simulink model "rull_stamp_hiv_modell"  (R2022a)
settings: Solver=VariableStepAuto  StartTime=0.0  StopTime=30  RelTol=1e-3
values from neighbouring files (symbols this model uses):
  A_topp = 0.286615    [Modell_verdier.m]
  B_r_t = 0.000799434    [Modell_verdier.m]
  B_s_f = 0.002833197    [Modell_verdier.m]
  B_s_t = 0.000183411    [Modell_verdier.m]
  C_D = 1.28    [Modell_verdier.m]
  Fb = 226    [Modell_verdier.m]
  g = 9.81    [Modell_verdier.m]
  I_rull = 1.28294    [Modell_verdier.m]
  I_stamp = 1.29837    [Modell_verdier.m]
  masse = 22.49    [Modell_verdier.m]
  phi_motor_rull = deg2rad(90-61.7)    [Modell_verdier.m]
  r_Fb = 0.036    [Modell_verdier.m]
  r_motor_rull = 0.277    [Modell_verdier.m]
  r_motor_stamp = 0.269    [Modell_verdier.m]
  tetthet_vann = 1000    [Modell_verdier.m]
  theta_motor_stamp = deg2rad(90-60.8)    [Modell_verdier.m]
libraries: simulink_extras x6
settings Model: Creator=andre  LastModifiedBy=andre

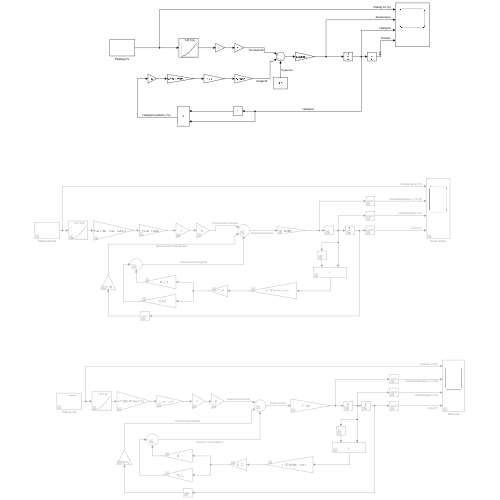
[thumbnail: Simulink's stored preview of the top-level diagram]
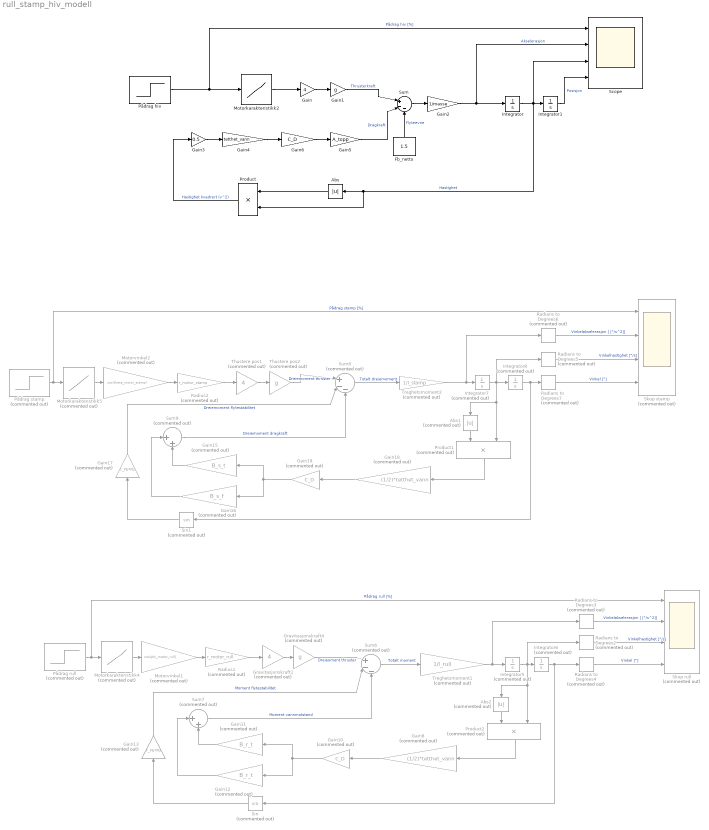
== system rull_stamp_hiv_modell ==
  Abs : Abs  SaturateOnIntegerOverflow=off
  Abs1 : Abs  Commented=on  SaturateOnIntegerOverflow=off
  Abs2 : Abs  Commented=on  SaturateOnIntegerOverflow=off
  Fb_netto : Constant  Value=1.5
  Gain : Gain  Gain=4
  Gain1 : Gain  Gain=g
  Gain10 : Gain  Commented=on  Gain=C_D
  Gain11 : Gain  Commented=on  Gain=B_r_t
  Gain12 : Gain  Commented=on  Gain=B_r_t
  Gain13 : Gain  Commented=on  Gain=r_Fb*Fb
  Gain15 : Gain  Commented=on  Gain=B_s_t
  Gain16 : Gain  Commented=on  Gain=B_s_f
  Gain17 : Gain  Commented=on  Gain=r_Fb*Fb
  Gain18 : Gain  Commented=on  Gain=(1/2)*tetthet_vann
  Gain19 : Gain  Commented=on  Gain=C_D
  Gain2 : Gain  Gain=1/masse
  Gain3 : Gain  Gain=0.5
  Gain4 : Gain  Gain=tetthet_vann
  Gain5 : Gain  Gain=A_topp
  Gain6 : Gain  Gain=C_D
  Gain8 : Gain  Commented=on  Gain=(1/2)*tetthet_vann
  Gravitasjonskraft1 : Gain  Commented=on  Gain=4
  Gravitasjonskraft4 : Gain  Commented=on  Gain=g
  Integrator : Integrator
  Integrator1 : Integrator  InitialCondition=0.5
  Integrator5 : Integrator  Commented=on
  Integrator6 : Integrator  Commented=on  InitialCondition=pi/4
  Integrator7 : Integrator  Commented=on
  Integrator8 : Integrator  Commented=on  InitialCondition=pi/4
  Motorkarakteristikk2 : Lookup_n-D  NumberOfTableDimensions=1  BreakpointsForDimension1="[0   12.5000   25.0000   37.5000   50.0000   62.5000   75.0000   87.5000  100.0000]"  Table=[0 0.1403 0.2807 0.5874 0.8942 1.3908 1.8874 2.3507 2.8140]  InternalRulePriority=Speed  RndMeth=Simplest
  Motorkarakteristikk4 : Lookup_n-D  Commented=on  NumberOfTableDimensions=1  BreakpointsForDimension1="[0   12.5000   25.0000   37.5000   50.0000   62.5000   75.0000   87.5000  100.0000]"  Table="[0    0.0370    0.2589    0.5675    0.8927    1.2590    1.7264    2.2152    2.7880]"  InternalRulePriority=Speed  RndMeth=Simplest
  Motorkarakteristikk5 : Lookup_n-D  Commented=on  NumberOfTableDimensions=1  BreakpointsForDimension1="[0   12.5000   25.0000   37.5000   50.0000   62.5000   75.0000   87.5000  100.0000]"  Table="[0    0.0370    0.2589    0.5675    0.8927    1.2590    1.7264    2.2152    2.7880]"  InternalRulePriority=Speed  RndMeth=Simplest
  Motorvinkel1 : Gain  Commented=on  Gain=cos(phi_motor_rull)
  Motorvinkel2 : Gain  Commented=on  Gain=cos(theta_motor_stamp)
  Product : Product
  Product1 : Product  Commented=on
  Product2 : Product  Commented=on
  Pådrag hiv : Step  Time=3  After=50  SampleTime=0
  Pådrag rull : Step  Commented=on  Time=10  After=30  SampleTime=0
  Pådrag stamp : Step  Commented=on  Time=10  After=30  SampleTime=0
  Radians to Degrees{2..7} (6 alike) : simulink_extras/Transformations/Radians to Degrees  Commented=on
  Radius1 : Gain  Commented=on  Gain=r_motor_rull
  Radius2 : Gain  Commented=on  Gain=r_motor_stamp
  Scope : Scope  NumInputPorts=4
  Sin : Trigonometry  Commented=on
  Sin1 : Trigonometry  Commented=on
  Skop rull : Scope  Commented=on  NumInputPorts=4
  Skop stamp : Scope  Commented=on  NumInputPorts=4
  Sum : Sum  Inputs=|+--
  Sum6 : Sum  Commented=on  Inputs=|+--
  Sum7 : Sum  Commented=on  Inputs=|++
  Sum8 : Sum  Commented=on  Inputs=|+--
  Sum9 : Sum  Commented=on  Inputs=|++
  Thustere pos1 : Gain  Commented=on  Gain=4
  Thustere pos2 : Gain  Commented=on  Gain=g
  Treghetsmoment1 : Gain  Commented=on  Gain=1/I_rull
  Treghetsmoment2 : Gain  Commented=on  Gain=1/I_stamp
  wires:
  Gain/1 -> Gain1/1
  Gain1/1 -> Sum/1  "Thrusterkraft"
  Sum/1 -> Gain2/1
  Gain2/1 -> Integrator/1, Scope/2  "Akselerasjon"
  Integrator/1 -> Integrator1/1, Product/2, Abs/1, Scope/3  "Hastighet"
  Abs/1 -> Product/1
  Product/1 -> Gain3/1  "Hastighet kvadrert (v^2)"
  Gain3/1 -> Gain4/1
  Gain4/1 -> Gain6/1
  Gain6/1 -> Gain5/1
  Gain5/1 -> Sum/2  "Dragkraft"
  Fb_netto/1 -> Sum/3  "Flyteevne"
  Pådrag hiv/1 -> Scope/1, Motorkarakteristikk2/1  "Pådrag hiv [%]"
  Motorkarakteristikk2/1 -> Gain/1
  Integrator1/1 -> Scope/4  "Posisjon"
  Motorkarakteristikk5/1 -> Motorvinkel2/1
  Abs1/1 -> Product1/1
  Sum8/1 -> Treghetsmoment2/1  "Totalt dreiemoment"
  Product1/1 -> Gain18/1
  Integrator8/1 -> Sin1/1, Radians to Degrees7/1
  Treghetsmoment2/1 -> Radians to Degrees6/1, Integrator7/1
  Sin1/1 -> Gain17/1
  Integrator7/1 -> Radians to Degrees5/1, Abs1/1, Product1/2, Integrator8/1
  Gain15/1 -> Sum9/2
  Radius2/1 -> Thustere pos1/1
  Radians to Degrees7/1 -> Skop stamp/4  "Vinkel [°]"
  Radians to Degrees5/1 -> Skop stamp/3  "Vinkelhastighet [°/s]"
  Gain16/1 -> Sum9/1
  Sum9/1 -> Sum8/3  "Dreiemoment dragkraft"
  Motorvinkel2/1 -> Radius2/1
  Radians to Degrees6/1 -> Skop stamp/2  "Vinkelakselerasjon [ [°/s^2]]"
  Pådrag stamp/1 -> Skop stamp/1, Motorkarakteristikk5/1  "Pådrag stamp [%]"
  Thustere pos1/1 -> Thustere pos2/1
  Thustere pos2/1 -> Sum8/1  "Dreiemoment thruster"
  Gain18/1 -> Gain19/1
  Gain19/1 -> Gain15/1, Gain16/1
  Gain17/1 -> Sum8/2  "Dreiemoment flytestabilitet"
  Gain11/1 -> Sum7/2
  Gain8/1 -> Gain10/1
  Radians to Degrees2/1 -> Skop rull/3  "Vinkelhastighet [°/s]"
  Treghetsmoment1/1 -> Radians to Degrees3/1, Integrator5/1
  Pådrag rull/1 -> Motorkarakteristikk4/1, Skop rull/1  "Pådrag rull [%]"
  Gain10/1 -> Gain12/1, Gain11/1
  Integrator5/1 -> Abs2/1, Product2/2, Integrator6/1, Radians to Degrees2/1
  Gravitasjonskraft4/1 -> Sum6/1  "Dreieoment thruster"
  Abs2/1 -> Product2/1
  Sin/1 -> Gain13/1
  Radians to Degrees3/1 -> Skop rull/2  "Vinkelakselerasjon [ [°/s^2]]"
  Integrator6/1 -> Sin/1, Radians to Degrees4/1
  Sum6/1 -> Treghetsmoment1/1  "Totalt moment"
  Radians to Degrees4/1 -> Skop rull/4  "Vinkel [°]"
  Product2/1 -> Gain8/1
  Motorvinkel1/1 -> Radius1/1
  Motorkarakteristikk4/1 -> Motorvinkel1/1
  Gain12/1 -> Sum7/1
  Sum7/1 -> Sum6/3  "Moment vannmotstand"
  Gain13/1 -> Sum6/2  "Moment flytestabilitet"
  Radius1/1 -> Gravitasjonskraft1/1
  Gravitasjonskraft1/1 -> Gravitasjonskraft4/1
